simulink model "model"  (R2020b)
settings: Solver=VariableStepAuto  StartTime=0.0  StopTime=35  RelTol=1e-3
undefined symbols (not defined in the file): A, B, R, S, T, Ts
libraries: simulink x1
settings Model: Creator=hrvoje  LastModifiedBy=hrvoje

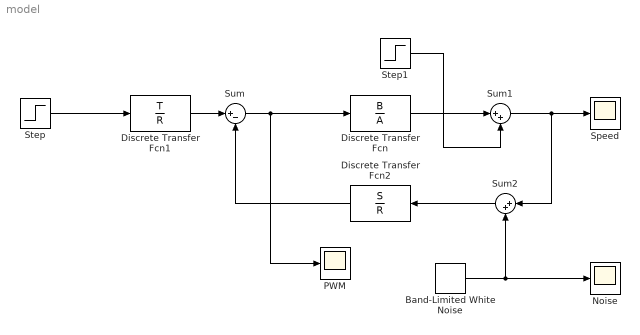
== system model ==
  Band-Limited White Noise : simulink/Sources/Band-Limited White Noise  Cov=[0.05]  Ts=Ts  seed=[23341]
  Discrete Transfer Fcn : DiscreteTransferFcn  Numerator=B  Denominator=A
  Discrete Transfer Fcn1 : DiscreteTransferFcn  Numerator=T  Denominator=R
  Discrete Transfer Fcn2 : DiscreteTransferFcn  Numerator=S  Denominator=R
  Noise : Scope
  PWM : Scope
  Speed : Scope
  Step : Step  Time=5  After=20  SampleTime=Ts
  Step1 : Step  Time=15  After=-5  SampleTime=Ts
  Sum : Sum  Inputs=|+-
  Sum1 : Sum  Inputs=|++
  Sum2 : Sum  Inputs=|++
  wires:
  Discrete Transfer Fcn1/1 -> Sum/1
  Discrete Transfer Fcn2/1 -> Sum/2
  Sum2/1 -> Discrete Transfer Fcn2/1
  Band-Limited White Noise/1 -> Sum2/2, Noise/1
  Sum/1 -> Discrete Transfer Fcn/1, PWM/1
  Discrete Transfer Fcn/1 -> Sum1/1
  Sum1/1 -> Sum2/1, Speed/1
  Step1/1 -> Sum1/2
  Step/1 -> Discrete Transfer Fcn1/1
